simulink model "MEGN544controlsHW_NickTaylor_MODEL"  (R2023b)
settings: Solver=VariableStepAuto  StartTime=0.0  StopTime=10.0  RelTol=1e-3
settings Model: Creator=Iris Fuqyu  LastModifiedBy=Iris Fuqyu

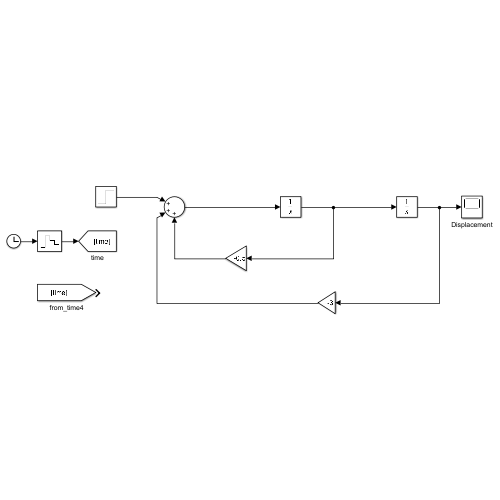
[thumbnail: Simulink's stored preview of the top-level diagram]
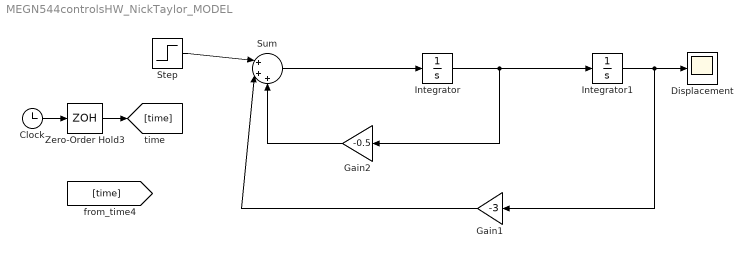
== system MEGN544controlsHW_NickTaylor_MODEL ==
  Clock : Clock
  Displacement : Scope
  Gain1 : Gain  Gain=-3
  Gain2 : Gain  Gain=-0.5
  Integrator : Integrator
  Integrator1 : Integrator
  Step : Step  SampleTime=0
  Sum : Sum  Inputs=|+++
  Zero-Order Hold3 : ZeroOrderHold  SampleTime=0.001
  wires:
  Clock/1 -> Zero-Order Hold3/1
  Zero-Order Hold3/1 -> [time]
  Step/1 -> Sum/1
  Gain1/1 -> Sum/2
  Gain2/1 -> Sum/3
  Sum/1 -> Integrator/1
  Integrator1/1 -> Gain1/1, Displacement/1
  Integrator/1 -> Gain2/1, Integrator1/1
